simulink model "thermalBuilding3211"  (Simulink 8.3)
settings: Solver=ode5  StartTime=0.0  StopTime=24  FixedStep=stepSize  RelTol=1e-3
model workspace: external: MAT-File D:\PROGRAMMING-IDEs\MATLAB\1WORKSPACE\1_Projects\Smart-Building\WIN/Data/wsVars/thermalBuilding3211WS.mat (data not in the file)
undefined symbols (not defined in the file): Ca, Ceq, cost, DiscIntNeverNeededParam, Mafc, Mafh, Req, Rwall, stepSize, TAout, TCooler, THeater, TInit, TSet1, TSet2, TSet3
libraries: dspsigops x1
(part 2 of 2)

== system thermalBuilding3211/HVAC System/Cooler1/F2C   converter1 ==
  F : Inport
  Constant : Constant  Value=32  OutDataTypeStr=Inherit: Inherit via back propagation
  Gain1 : Gain  Gain=5/9  SaturateOnIntegerOverflow=on  OutDataTypeStr=Inherit: Same as input  ParamDataTypeStr=Inherit: Same as input
  Sum : Sum  Inputs=+-  SaturateOnIntegerOverflow=on  InputSameDT=on  OutDataTypeStr=Inherit: Same as first input
  C : Outport
  wires:
  Constant/1 -> Sum/2
  Gain1/1 -> C/1
  Sum/1 -> Gain1/1
  F/1 -> Sum/1

== system thermalBuilding3211/HVAC System/Cooler2/F2C   converter1 ==
  F : Inport
  Constant : Constant  Value=32  OutDataTypeStr=Inherit: Inherit via back propagation
  Gain1 : Gain  Gain=5/9  SaturateOnIntegerOverflow=on  OutDataTypeStr=Inherit: Same as input  ParamDataTypeStr=Inherit: Same as input
  Sum : Sum  Inputs=+-  SaturateOnIntegerOverflow=on  InputSameDT=on  OutDataTypeStr=Inherit: Same as first input
  C : Outport
  wires:
  Constant/1 -> Sum/2
  Gain1/1 -> C/1
  Sum/1 -> Gain1/1
  F/1 -> Sum/1

== system thermalBuilding3211/HVAC System/Cooler3/F2C   converter1 ==
  F : Inport
  Constant : Constant  Value=32  OutDataTypeStr=Inherit: Inherit via back propagation
  Gain1 : Gain  Gain=5/9  SaturateOnIntegerOverflow=on  OutDataTypeStr=Inherit: Same as input  ParamDataTypeStr=Inherit: Same as input
  Sum : Sum  Inputs=+-  SaturateOnIntegerOverflow=on  InputSameDT=on  OutDataTypeStr=Inherit: Same as first input
  C : Outport
  wires:
  Constant/1 -> Sum/2
  Gain1/1 -> C/1
  Sum/1 -> Gain1/1
  F/1 -> Sum/1

== system thermalBuilding3211/HVAC System/Heater1/F2C   converter1 ==
  F : Inport
  Constant : Constant  Value=32  OutDataTypeStr=Inherit: Inherit via back propagation
  Gain1 : Gain  Gain=5/9  SaturateOnIntegerOverflow=on  OutDataTypeStr=Inherit: Same as input  ParamDataTypeStr=Inherit: Same as input
  Sum : Sum  Inputs=+-  SaturateOnIntegerOverflow=on  InputSameDT=on  OutDataTypeStr=Inherit: Same as first input
  C : Outport
  wires:
  Constant/1 -> Sum/2
  Gain1/1 -> C/1
  Sum/1 -> Gain1/1
  F/1 -> Sum/1

== system thermalBuilding3211/HVAC System/Heater2/F2C   converter1 ==
  F : Inport
  Constant : Constant  Value=32  OutDataTypeStr=Inherit: Inherit via back propagation
  Gain1 : Gain  Gain=5/9  SaturateOnIntegerOverflow=on  OutDataTypeStr=Inherit: Same as input  ParamDataTypeStr=Inherit: Same as input
  Sum : Sum  Inputs=+-  SaturateOnIntegerOverflow=on  InputSameDT=on  OutDataTypeStr=Inherit: Same as first input
  C : Outport
  wires:
  Constant/1 -> Sum/2
  Gain1/1 -> C/1
  Sum/1 -> Gain1/1
  F/1 -> Sum/1

== system thermalBuilding3211/HVAC System/Heater3/F2C   converter1 ==
  F : Inport
  Constant : Constant  Value=32  OutDataTypeStr=Inherit: Inherit via back propagation
  Gain1 : Gain  Gain=5/9  SaturateOnIntegerOverflow=on  OutDataTypeStr=Inherit: Same as input  ParamDataTypeStr=Inherit: Same as input
  Sum : Sum  Inputs=+-  SaturateOnIntegerOverflow=on  InputSameDT=on  OutDataTypeStr=Inherit: Same as first input
  C : Outport
  wires:
  Constant/1 -> Sum/2
  Gain1/1 -> C/1
  Sum/1 -> Gain1/1
  F/1 -> Sum/1

== system thermalBuilding3211/Building/Room1/Controller1/Reference Temperature ==
  F2C   converter1 : Subsystem  mask(F2C){}
      mask help:
      | Conversion from degrees Fahrenheit to degrees Celsius.
      |
      | C = (F-32) * (5/9);
      mask Display: image(imread('celsius.jpg'))
  Set Point : Constant  Value=TSet1
  Tset : Outport
  wires:
  Set Point/1 -> F2C   converter1/1(F)
  F2C   converter1/1(C) -> Tset/1

== system thermalBuilding3211/Building/Room1/Controller1/RoC1 ==
  In1 : Inport
  Constant1 : Constant  Value=TInit
  Constant2 : Constant  Value=0
  F2C   converter1 : Subsystem  mask(F2C){}
      mask help:
      | Conversion from degrees Fahrenheit to degrees Celsius.
      |
      | C = (F-32) * (5/9);
      mask Display: image(imread('celsius.jpg'))
  Memory1 : Memory
  Multiport Switch1 : MultiPortSwitch  DataPortOrder=Specify indices  Inputs=2  DataPortIndices={1,0}  DiagnosticForDefault=None
  Relational Operator : RelationalOperator  Operator===  OutDataTypeStr=boolean
  Subtract : Sum  Inputs=+-
  Out1 : Outport
  wires:
  Constant1/1 -> F2C   converter1/1(F)
  Relational Operator/1 -> Multiport Switch1/1
  Constant2/1 -> Multiport Switch1/2
  Multiport Switch1/1 -> Out1/1
  Memory1/1 -> Subtract/2
  F2C   converter1/1(C) -> Relational Operator/1
  In1/1 -> Memory1/1, Subtract/1
  Subtract/1 -> Multiport Switch1/3, Relational Operator/2

== system thermalBuilding3211/Building/Room1/SystemOut1/C2F converter1 ==
  F : Inport
  Constant1 : Constant  Value=32  OutDataTypeStr=Inherit: Inherit via back propagation
  Gain : Gain  Gain=9/5  SaturateOnIntegerOverflow=on  OutDataTypeStr=Inherit: Same as input  ParamDataTypeStr=Inherit: Same as input
  Sum1 : Sum  SaturateOnIntegerOverflow=on  InputSameDT=on  OutDataTypeStr=Inherit: Same as first input
  C : Outport
  wires:
  F/1 -> Gain/1
  Gain/1 -> Sum1/1
  Sum1/1 -> C/1
  Constant1/1 -> Sum1/2

== system thermalBuilding3211/Building/Room1/SystemOut1/C2F converter2 ==
  F : Inport
  Constant1 : Constant  Value=32  OutDataTypeStr=Inherit: Inherit via back propagation
  Gain : Gain  Gain=9/5  SaturateOnIntegerOverflow=on  OutDataTypeStr=Inherit: Same as input  ParamDataTypeStr=Inherit: Same as input
  Sum1 : Sum  SaturateOnIntegerOverflow=on  InputSameDT=on  OutDataTypeStr=Inherit: Same as first input
  C : Outport
  wires:
  Constant1/1 -> Sum1/2
  Sum1/1 -> C/1
  Gain/1 -> Sum1/1
  F/1 -> Gain/1

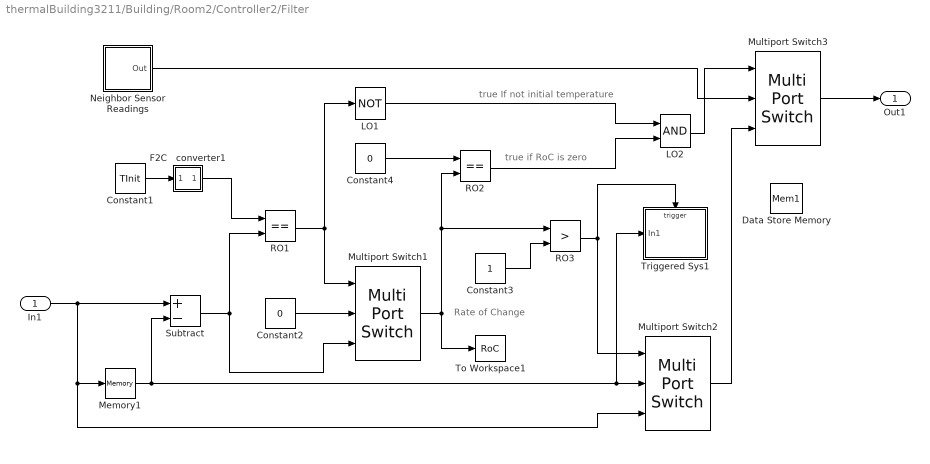
== system thermalBuilding3211/Building/Room2/Controller2/Filter ==
  note: true if RoC is zero
  note: true If not initial temperature
  note: Rate of Change
  In1 : Inport
  Constant1 : Constant  Value=TInit
  Constant2 : Constant  Value=0
  Constant3 : Constant
  Constant4 : Constant  Value=0
  Data Store Memory : DataStoreMemory  DataStoreName=Mem1  ReadBeforeWriteMsg=warning  WriteAfterWriteMsg=warning  WriteAfterReadMsg=warning
  F2C   converter1 : Subsystem  mask(F2C){}
      mask help:
      | Conversion from degrees Fahrenheit to degrees Celsius.
      |
      | C = (F-32) * (5/9);
      mask Display: image(imread('celsius.jpg'))
  LO1 : Logic  Operator=NOT  IconShape=distinctive  AllPortsSameDT=off  OutDataTypeStr=boolean
  LO2 : Logic  AllPortsSameDT=off  OutDataTypeStr=boolean
  Memory1 : Memory
  Multiport Switch1 : MultiPortSwitch  DataPortOrder=Specify indices  Inputs=2  DataPortIndices={1,0}  DiagnosticForDefault=None
  Multiport Switch2 : MultiPortSwitch  DataPortOrder=Specify indices  Inputs=2  DataPortIndices={1,0}  DiagnosticForDefault=None
  Multiport Switch3 : MultiPortSwitch  DataPortOrder=Specify indices  Inputs=2  DataPortIndices={1,0}  DiagnosticForDefault=None
  Neighbor Sensor Readings : Subsystem
  RO1 : RelationalOperator  Operator===  OutDataTypeStr=boolean
  RO2 : RelationalOperator  Operator===  OutDataTypeStr=boolean
  RO3 : RelationalOperator  Operator=>  OutDataTypeStr=boolean
  Subtract : Sum  Inputs=+-
  To Workspace1 : ToWorkspace  VariableName=RoC  SampleTime=-1
  Triggered Sys1 : Subsystem  TreatAsAtomicUnit=on
  Out1 : Outport
  wires:
  Constant1/1 -> F2C   converter1/1(F)
  RO1/1 -> LO1/1, Multiport Switch1/1
  Constant2/1 -> Multiport Switch1/2
  Multiport Switch1/1 -> RO2/2, RO3/1, To Workspace1/1
  RO3/1 -> Multiport Switch2/1, Triggered Sys1/Trigger
  Constant3/1 -> RO3/2
  Multiport Switch2/1 -> Multiport Switch3/3
  Memory1/1 -> Triggered Sys1/1(In1), Multiport Switch2/2, Subtract/2
  F2C   converter1/1(C) -> RO1/1
  In1/1 -> Multiport Switch2/3, Memory1/1, Subtract/1
  Subtract/1 -> RO1/2, Multiport Switch1/3
  LO1/1 -> LO2/1
  LO2/1 -> Multiport Switch3/1
  RO2/1 -> LO2/2
  Constant4/1 -> RO2/1
  Multiport Switch3/1 -> Out1/1
  Neighbor Sensor Readings/1(Out) -> Multiport Switch3/2

== system thermalBuilding3211/Building/Room2/Controller2/Reference Temperature ==
  F2C   converter1 : Subsystem  mask(F2C){}
      mask help:
      | Conversion from degrees Fahrenheit to degrees Celsius.
      |
      | C = (F-32) * (5/9);
      mask Display: image(imread('celsius.jpg'))
  Set Point : Constant  Value=TSet2
  Tset : Outport
  wires:
  Set Point/1 -> F2C   converter1/1(F)
  F2C   converter1/1(C) -> Tset/1

== system thermalBuilding3211/Building/Room2/Controller2/RoC2 ==
  In1 : Inport
  Constant1 : Constant  Value=TInit
  Constant2 : Constant  Value=0
  F2C   converter1 : Subsystem  mask(F2C){}
      mask help:
      | Conversion from degrees Fahrenheit to degrees Celsius.
      |
      | C = (F-32) * (5/9);
      mask Display: image(imread('celsius.jpg'))
  Memory1 : Memory
  Multiport Switch1 : MultiPortSwitch  DataPortOrder=Specify indices  Inputs=2  DataPortIndices={1,0}  DiagnosticForDefault=None
  Relational Operator : RelationalOperator  Operator===  OutDataTypeStr=boolean
  Subtract : Sum  Inputs=+-
  Out1 : Outport
  wires:
  Constant1/1 -> F2C   converter1/1(F)
  Relational Operator/1 -> Multiport Switch1/1
  Constant2/1 -> Multiport Switch1/2
  Multiport Switch1/1 -> Out1/1
  Memory1/1 -> Subtract/2
  F2C   converter1/1(C) -> Relational Operator/1
  In1/1 -> Memory1/1, Subtract/1
  Subtract/1 -> Multiport Switch1/3, Relational Operator/2

== system thermalBuilding3211/Building/Room2/SystemOut2/C2F converter1 ==
  F : Inport
  Constant1 : Constant  Value=32  OutDataTypeStr=Inherit: Inherit via back propagation
  Gain : Gain  Gain=9/5  SaturateOnIntegerOverflow=on  OutDataTypeStr=Inherit: Same as input  ParamDataTypeStr=Inherit: Same as input
  Sum1 : Sum  SaturateOnIntegerOverflow=on  InputSameDT=on  OutDataTypeStr=Inherit: Same as first input
  C : Outport
  wires:
  F/1 -> Gain/1
  Gain/1 -> Sum1/1
  Sum1/1 -> C/1
  Constant1/1 -> Sum1/2

== system thermalBuilding3211/Building/Room2/SystemOut2/C2F converter2 ==
  F : Inport
  Constant1 : Constant  Value=32  OutDataTypeStr=Inherit: Inherit via back propagation
  Gain : Gain  Gain=9/5  SaturateOnIntegerOverflow=on  OutDataTypeStr=Inherit: Same as input  ParamDataTypeStr=Inherit: Same as input
  Sum1 : Sum  SaturateOnIntegerOverflow=on  InputSameDT=on  OutDataTypeStr=Inherit: Same as first input
  C : Outport
  wires:
  Constant1/1 -> Sum1/2
  Sum1/1 -> C/1
  Gain/1 -> Sum1/1
  F/1 -> Gain/1

== system thermalBuilding3211/Building/Room2/Temperature Sensor2/Sample & Hold ==
  In1 : Inport
  In2 : Inport  Port=2
  In3 : Inport  Port=3
  Constant : Constant  Value=0
  LO : Logic  AllPortsSameDT=off  OutDataTypeStr=boolean
  Lower_Bound1 : RelationalOperator  Operator=~=  OutDataTypeStr=boolean
  RO : RelationalOperator  Operator=<  OutDataTypeStr=boolean
  Subtract : Sum  Inputs=-+
  Out1 : Outport
  wires:
  RO/1 -> LO/2
  Constant/1 -> Lower_Bound1/2
  In2/1 -> Subtract/2
  In3/1 -> RO/2
  Lower_Bound1/1 -> LO/1
  Subtract/1 -> RO/1
  In1/1 -> Subtract/1, Lower_Bound1/1
  LO/1 -> Out1/1

== system thermalBuilding3211/Building/Room2/Temperature Sensor2/Save time ==
  trigger : Inport
  time() : Inport  Port=2
  Clock_Count1 : Integrator  ExternalReset=rising  InitialConditionSource=external
  Constant1 : Constant  Value=0
  DTC1 : DataTypeConversion  OutMin=[1]  OutMax=[2]  OutDataTypeStr=double  ConvertRealWorld=Stored Integer (SI)
  t : Outport
  wires:
  time()/1 -> Clock_Count1/3
  Clock_Count1/1 -> DTC1/1
  Constant1/1 -> Clock_Count1/1
  trigger/1 -> Clock_Count1/2
  DTC1/1 -> t/1

== system thermalBuilding3211/Building/Room2/Temperature Sensor2/Single-Sample-Spike ==
  Constant1 : Constant  Value=0
  Memory : Memory
  Multiport Switch1 : MultiPortSwitch  DataPortOrder=Specify indices  Inputs=2  DataPortIndices={1,0}  DiagnosticForDefault=None
  Relational Operator1 : RelationalOperator  Operator=<  OutDataTypeStr=boolean
  Spike Probability : Constant  Value=stepSize*5/10
  Spike magnitude  (Celcius) : Constant  Value=7
  Spike Generator : MATLAB Function  TreatAsAtomicUnit=on
  Out : Outport
  wires:
  Spike Probability/1 -> Spike Generator/2(u2)
  Memory/1 -> Relational Operator1/1
  Spike Generator/1(y) -> Memory/1, Relational Operator1/2, Multiport Switch1/2
  Constant1/1 -> Multiport Switch1/3
  Multiport Switch1/1 -> Out/1
  Spike magnitude  (Celcius)/1 -> Spike Generator/1(u1)
  Relational Operator1/1 -> Multiport Switch1/1

== system thermalBuilding3211/Building/Room2/Temperature Sensor2/Timer ==
  Constant : Constant  Value=1/stepSize
  Constant1 : Constant
  Discrete-Time Integrator : DiscreteIntegrator  SampleTime=stepSize  ICPrevOutput=DiscIntNeverNeededParam  ICPrevScaledInput=DiscIntNeverNeededParam
  Product : Product
  Scope : Scope
  time() : Outport
  wires:
  Discrete-Time Integrator/1 -> Scope/1, Product/1
  Constant1/1 -> Discrete-Time Integrator/1
  Constant/1 -> Product/2
  Product/1 -> time()/1

== system thermalBuilding3211/Building/Room3/Controller3/Reference Temperature ==
  F2C   converter1 : Subsystem  mask(F2C){}
      mask help:
      | Conversion from degrees Fahrenheit to degrees Celsius.
      |
      | C = (F-32) * (5/9);
      mask Display: image(imread('celsius.jpg'))
  Set Point : Constant  Value=TSet3
  Tset : Outport
  wires:
  Set Point/1 -> F2C   converter1/1(F)
  F2C   converter1/1(C) -> Tset/1

== system thermalBuilding3211/Building/Room3/Controller3/RoC3 ==
  In1 : Inport
  Constant1 : Constant  Value=TInit
  Constant2 : Constant  Value=0
  F2C   converter1 : Subsystem  mask(F2C){}
      mask help:
      | Conversion from degrees Fahrenheit to degrees Celsius.
      |
      | C = (F-32) * (5/9);
      mask Display: image(imread('celsius.jpg'))
  Memory1 : Memory
  Multiport Switch1 : MultiPortSwitch  DataPortOrder=Specify indices  Inputs=2  DataPortIndices={1,0}  DiagnosticForDefault=None
  Relational Operator : RelationalOperator  Operator===  OutDataTypeStr=boolean
  Subtract : Sum  Inputs=+-
  Out1 : Outport
  wires:
  Constant1/1 -> F2C   converter1/1(F)
  Relational Operator/1 -> Multiport Switch1/1
  Constant2/1 -> Multiport Switch1/2
  Multiport Switch1/1 -> Out1/1
  Memory1/1 -> Subtract/2
  F2C   converter1/1(C) -> Relational Operator/1
  In1/1 -> Memory1/1, Subtract/1
  Subtract/1 -> Multiport Switch1/3, Relational Operator/2

== system thermalBuilding3211/Building/Room1/Controller1/Reference Temperature/F2C   converter1 ==
  F : Inport
  Constant : Constant  Value=32  OutDataTypeStr=Inherit: Inherit via back propagation
  Gain1 : Gain  Gain=5/9  SaturateOnIntegerOverflow=on  OutDataTypeStr=Inherit: Same as input  ParamDataTypeStr=Inherit: Same as input
  Sum : Sum  Inputs=+-  SaturateOnIntegerOverflow=on  InputSameDT=on  OutDataTypeStr=Inherit: Same as first input
  C : Outport
  wires:
  Constant/1 -> Sum/2
  Gain1/1 -> C/1
  Sum/1 -> Gain1/1
  F/1 -> Sum/1

== system thermalBuilding3211/Building/Room1/Controller1/RoC1/F2C   converter1 ==
  F : Inport
  Constant : Constant  Value=32  OutDataTypeStr=Inherit: Inherit via back propagation
  Gain1 : Gain  Gain=5/9  SaturateOnIntegerOverflow=on  OutDataTypeStr=Inherit: Same as input  ParamDataTypeStr=Inherit: Same as input
  Sum : Sum  Inputs=+-  SaturateOnIntegerOverflow=on  InputSameDT=on  OutDataTypeStr=Inherit: Same as first input
  C : Outport
  wires:
  Constant/1 -> Sum/2
  Gain1/1 -> C/1
  Sum/1 -> Gain1/1
  F/1 -> Sum/1

== system thermalBuilding3211/Building/Room2/Controller2/Filter/F2C   converter1 ==
  F : Inport
  Constant : Constant  Value=32  OutDataTypeStr=Inherit: Inherit via back propagation
  Gain1 : Gain  Gain=5/9  SaturateOnIntegerOverflow=on  OutDataTypeStr=Inherit: Same as input  ParamDataTypeStr=Inherit: Same as input
  Sum : Sum  Inputs=+-  SaturateOnIntegerOverflow=on  InputSameDT=on  OutDataTypeStr=Inherit: Same as first input
  C : Outport
  wires:
  Constant/1 -> Sum/2
  Gain1/1 -> C/1
  Sum/1 -> Gain1/1
  F/1 -> Sum/1

== system thermalBuilding3211/Building/Room2/Controller2/Filter/Neighbor Sensor Readings ==
  Add : Sum
  C2F converter1 : Subsystem  mask(F2C){}
      mask help:
      | Conversion from degrees Fahrenheit to degrees Celsius.
      |
      | F = C * (9/5) + 32;
      mask Display: image(imread('fahrenheit.jpg'))
  C2F converter2 : Subsystem  mask(F2C){}
      mask help:
      | Conversion from degrees Fahrenheit to degrees Celsius.
      |
      | F = C * (9/5) + 32;
      mask Display: image(imread('fahrenheit.jpg'))
  C2F converter3 : Subsystem  mask(F2C){}
      mask help:
      | Conversion from degrees Fahrenheit to degrees Celsius.
      |
      | F = C * (9/5) + 32;
      mask Display: image(imread('fahrenheit.jpg'))
  Constant1 : Constant  Value=2
  Data Store Read1 : DataStoreRead  DataStoreName=Tr1
  Data Store Read2 : DataStoreRead  DataStoreName=Tr3
  Divide : Product  Inputs=*/
  To Workspace : ToWorkspace  VariableName=Tr1  SampleTime=-1
  To Workspace1 : ToWorkspace  VariableName=Tr3  SampleTime=-1
  To Workspace2 : ToWorkspace  VariableName=Tr2  SampleTime=-1
  Out : Outport
  wires:
  Constant1/1 -> Divide/2
  Data Store Read1/1 -> Out/1, Add/1, C2F converter2/1(F)
  Data Store Read2/1 -> C2F converter3/1(F), Add/2
  Add/1 -> Divide/1
  Divide/1 -> C2F converter1/1(F)
  C2F converter1/1(C) -> To Workspace2/1
  C2F converter2/1(C) -> To Workspace/1
  C2F converter3/1(C) -> To Workspace1/1

== system thermalBuilding3211/Building/Room2/Controller2/Filter/Triggered Sys1 ==
  In1 : Inport
  Trigger : TriggerPort
  Data Store Write : DataStoreWrite  DialogController=Simulink.DDGSource  DataStoreName=Mem1
  To Workspace1 : ToWorkspace  VariableName=Mem1  SampleTime=-1
  wires:
  In1/1 -> Data Store Write/1, To Workspace1/1

== system thermalBuilding3211/Building/Room2/Controller2/Reference Temperature/F2C   converter1 ==
  F : Inport
  Constant : Constant  Value=32  OutDataTypeStr=Inherit: Inherit via back propagation
  Gain1 : Gain  Gain=5/9  SaturateOnIntegerOverflow=on  OutDataTypeStr=Inherit: Same as input  ParamDataTypeStr=Inherit: Same as input
  Sum : Sum  Inputs=+-  SaturateOnIntegerOverflow=on  InputSameDT=on  OutDataTypeStr=Inherit: Same as first input
  C : Outport
  wires:
  Constant/1 -> Sum/2
  Gain1/1 -> C/1
  Sum/1 -> Gain1/1
  F/1 -> Sum/1

== system thermalBuilding3211/Building/Room2/Controller2/RoC2/F2C   converter1 ==
  F : Inport
  Constant : Constant  Value=32  OutDataTypeStr=Inherit: Inherit via back propagation
  Gain1 : Gain  Gain=5/9  SaturateOnIntegerOverflow=on  OutDataTypeStr=Inherit: Same as input  ParamDataTypeStr=Inherit: Same as input
  Sum : Sum  Inputs=+-  SaturateOnIntegerOverflow=on  InputSameDT=on  OutDataTypeStr=Inherit: Same as first input
  C : Outport
  wires:
  Constant/1 -> Sum/2
  Gain1/1 -> C/1
  Sum/1 -> Gain1/1
  F/1 -> Sum/1

== system thermalBuilding3211/Building/Room3/Controller3/Reference Temperature/F2C   converter1 ==
  F : Inport
  Constant : Constant  Value=32  OutDataTypeStr=Inherit: Inherit via back propagation
  Gain1 : Gain  Gain=5/9  SaturateOnIntegerOverflow=on  OutDataTypeStr=Inherit: Same as input  ParamDataTypeStr=Inherit: Same as input
  Sum : Sum  Inputs=+-  SaturateOnIntegerOverflow=on  InputSameDT=on  OutDataTypeStr=Inherit: Same as first input
  C : Outport
  wires:
  Constant/1 -> Sum/2
  Gain1/1 -> C/1
  Sum/1 -> Gain1/1
  F/1 -> Sum/1

== system thermalBuilding3211/Building/Room3/Controller3/RoC3/F2C   converter1 ==
  F : Inport
  Constant : Constant  Value=32  OutDataTypeStr=Inherit: Inherit via back propagation
  Gain1 : Gain  Gain=5/9  SaturateOnIntegerOverflow=on  OutDataTypeStr=Inherit: Same as input  ParamDataTypeStr=Inherit: Same as input
  Sum : Sum  Inputs=+-  SaturateOnIntegerOverflow=on  InputSameDT=on  OutDataTypeStr=Inherit: Same as first input
  C : Outport
  wires:
  Constant/1 -> Sum/2
  Gain1/1 -> C/1
  Sum/1 -> Gain1/1
  F/1 -> Sum/1

== system thermalBuilding3211/Building/Room2/Controller2/Filter/Neighbor Sensor Readings/C2F converter1 ==
  F : Inport
  Constant1 : Constant  Value=32  OutDataTypeStr=Inherit: Inherit via back propagation
  Gain : Gain  Gain=9/5  SaturateOnIntegerOverflow=on  OutDataTypeStr=Inherit: Same as input  ParamDataTypeStr=Inherit: Same as input
  Sum1 : Sum  SaturateOnIntegerOverflow=on  InputSameDT=on  OutDataTypeStr=Inherit: Same as first input
  C : Outport
  wires:
  F/1 -> Gain/1
  Gain/1 -> Sum1/1
  Sum1/1 -> C/1
  Constant1/1 -> Sum1/2

== system thermalBuilding3211/Building/Room2/Controller2/Filter/Neighbor Sensor Readings/C2F converter2 ==
  F : Inport
  Constant1 : Constant  Value=32  OutDataTypeStr=Inherit: Inherit via back propagation
  Gain : Gain  Gain=9/5  SaturateOnIntegerOverflow=on  OutDataTypeStr=Inherit: Same as input  ParamDataTypeStr=Inherit: Same as input
  Sum1 : Sum  SaturateOnIntegerOverflow=on  InputSameDT=on  OutDataTypeStr=Inherit: Same as first input
  C : Outport
  wires:
  Constant1/1 -> Sum1/2
  Sum1/1 -> C/1
  Gain/1 -> Sum1/1
  F/1 -> Gain/1

== system thermalBuilding3211/Building/Room2/Controller2/Filter/Neighbor Sensor Readings/C2F converter3 ==
  F : Inport
  Constant1 : Constant  Value=32  OutDataTypeStr=Inherit: Inherit via back propagation
  Gain : Gain  Gain=9/5  SaturateOnIntegerOverflow=on  OutDataTypeStr=Inherit: Same as input  ParamDataTypeStr=Inherit: Same as input
  Sum1 : Sum  SaturateOnIntegerOverflow=on  InputSameDT=on  OutDataTypeStr=Inherit: Same as first input
  C : Outport
  wires:
  F/1 -> Gain/1
  Gain/1 -> Sum1/1
  Sum1/1 -> C/1
  Constant1/1 -> Sum1/2

== matlab function Building/Room2/Temperature Sensor2/Single-Sample-Spike/Spike Generator ==
  data: u1 input double; y output double; u2 input double
function y = fcn(u1, u2)
%#codegen
coder.extrinsic('datasample');
coder.extrinsic('randsample');
% initialize y
y = 0;
% sampling
a = datasample([0 u1], 1, 'Weights', [1-u2 u2]);
b = randsample([0 u1], 1, true, [1-u2 u2]);
y = b;

end
